simulink model "Model_RLC_SS_14b"  (R2014b)
settings: Solver=ode45  StartTime=0.0  StopTime=10.0  RelTol=1e-3
undefined symbols (not defined in the file or in its folder): in, param
libraries: simulink x1
settings Model: Creator=Arek  LastModifiedBy=Arek

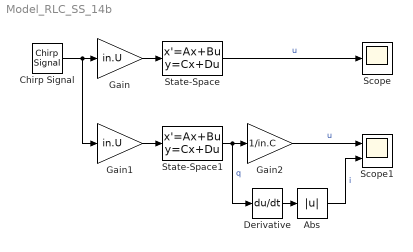
== system Model_RLC_SS_14b ==
  Abs : Abs
  Chirp Signal : simulink/Sources/Chirp Signal  f1=freq.fmin  T=param.tmax  f2=freq.fmax
  Derivative : Derivative
  Gain : Gain  Gain=in.U
  Gain1 : Gain  Gain=in.U
  Gain2 : Gain  Gain=1/in.C
  Scope : Scope
      settings: ShowLegends=on  YMin=-25  YMax=25
  Scope1 : Scope  NumInputPorts=2
      settings: ShowLegends=on  YMin=-5~-5  YMax=5~5
  State-Space : StateSpace  A=[-in.R/in.L -1/in.L;1/in.C 0]  B=[1/in.L; 0]  C=[0 1]  D=[0]  X0=param.ic
  State-Space1 : StateSpace  A=[-in.R/in.L -1/in.C;1/in.L 0]  B=[1; 0]  C=[0 1]  D=[0]  X0=param.ic
  wires:
  Gain/1 -> State-Space/1
  State-Space/1 -> Scope/1  "u"
  Chirp Signal/1 -> Gain1/1, Gain/1
  Gain1/1 -> State-Space1/1
  State-Space1/1 -> Derivative/1, Gain2/1  "q"
  Derivative/1 -> Abs/1
  Gain2/1 -> Scope1/1  "u"
  Abs/1 -> Scope1/2  "i"
